simulink model "model"  (R2017b)
settings: Solver=ode45  StartTime=0.0  StopTime=0.05  RelTol=1e-3  EnableMultiTasking=on
InitFcn:
  | Fs=100e3;
  | w=Fs*2*pi;
  | 
  | Vdc=100;
  | 
  | LP=200e-6;
  | LS=LP;
  | 
  | CP=1/w^2/LP;
  | CS=1/w^2/LS;
  | 
  | MPS=20e-6;
  | 
  | 
  | Rlp=0.1;
  | Rls=0.1;
undefined symbols (not defined in the file): LM, MPM, MSM, Rlm
libraries: powerlib x20, simulink x2, peRmsMeasurement x1
settings Model: Creator=User  LastModifiedBy=SuperWindows
settings DataIOCC: LimitDataPoints=on  SaveFormat=Array
settings OptimizationCC: LifeSpan=inf
settings DebuggingCC: SolverPrmCheckMsg=warning  SFUnexpectedBacktrackingDiag=warning  SFNoUnconditionalDefaultTransitionDiag=warning  SFExecutionAtInitializationDiag=none
settings HardwareCC: ProdBitPerPointer=32  ProdBitPerSizeT=32  ProdBitPerPtrDiffT=32  ProdLargestAtomicFloat=None  ProdIntDivRoundTo=Undefined  ProdEndianess=Unspecified  ProdWordSize=32  ProdHWDeviceType=32-bit Generic
settings ModelReferenceCC: PropagateSignalLabelsOutOfModel=off
settings CodeAppCC: StateflowObjectComments=on
settings GRTTargetCC: TargetLangStandard=C89/C90 (ANSI)  GeneratePreprocessorConditionals=Disable all
settings ConfigComp: CovMetricSettings=dw  CovHtmlReporting=on  CovSaveCumulativeToWorkspaceVar=on  CovSaveSingleToWorkspaceVar=on  CovExternalEMLEnable=off  CovSFcnEnable=off
settings SimscapeCC: SimscapeNormalizeSystem=off

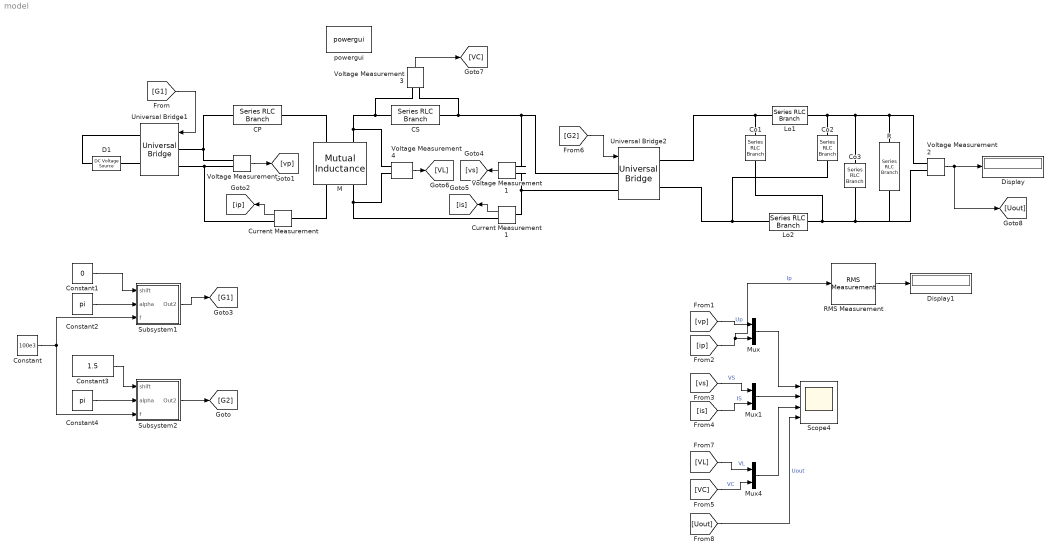
== system model ==
  CP : powerlib/Elements/Series RLC Branch  LConnTagsString=__new0  RConnTagsString=__new0  BranchType=C  Resistance=5  Inductance=1e-3  SetiL0=off  InitialCurrent=0  Capacitance=CP  Setx0=off  InitialVoltage=0  Measurements=Branch voltage
  CS : powerlib/Elements/Series RLC Branch  LConnTagsString=__new0  RConnTagsString=__new0  BranchType=C  Resistance=1  Inductance=1e-3  SetiL0=off  InitialCurrent=0  Capacitance=CS  Setx0=off  InitialVoltage=0  Measurements=Branch voltage
  Co1 : powerlib/Elements/Series RLC Branch  LConnTagsString=__new0  RConnTagsString=__new0  BranchType=C  Resistance=1  Inductance=1e-3  SetiL0=off  InitialCurrent=0  Capacitance=4700e-6  Setx0=on  InitialVoltage=60  Measurements=Branch voltage
  Co2 : powerlib/Elements/Series RLC Branch  LConnTagsString=__new0  RConnTagsString=__new0  BranchType=C  Resistance=1  Inductance=1e-3  SetiL0=off  InitialCurrent=0  Capacitance=4700e-6  Setx0=on  InitialVoltage=60  Measurements=Branch voltage
  Co3 : powerlib/Elements/Series RLC Branch  LConnTagsString=__new0  RConnTagsString=__new0  BranchType=C  Resistance=1  Inductance=1e-3  SetiL0=off  InitialCurrent=0  Capacitance=4700e-6  Setx0=on  InitialVoltage=60  Measurements=Branch voltage
  Constant : Constant  Value=100e3
  Constant1 : Constant  Value=0
  Constant2 : Constant  Value=pi
  Constant3 : Constant  Value=1.5
  Constant4 : Constant  Value=pi
  Current Measurement : powerlib/Measurements/Current Measurement  PhasorSimulation=off  OutputType=Complex  PSBequivalent=0
  Current Measurement1 : powerlib/Measurements/Current Measurement  PhasorSimulation=off  OutputType=Complex  PSBequivalent=0
  D1 : powerlib/Electrical Sources/DC Voltage Source  Amplitude=Vdc  Measurements=None
  Display : Display
  Display1 : Display
  Lo1 : powerlib/Elements/Series RLC Branch  LConnTagsString=__new0  RConnTagsString=__new0  BranchType=L  Resistance=1  Inductance=1e-3  SetiL0=off  InitialCurrent=0  Capacitance=4700e-6  Setx0=on  InitialVoltage=60  Measurements=Branch voltage
  Lo2 : powerlib/Elements/Series RLC Branch  LConnTagsString=__new0  RConnTagsString=__new0  BranchType=L  Resistance=1  Inductance=1e-3  SetiL0=off  InitialCurrent=0  Capacitance=4700e-6  Setx0=on  InitialVoltage=60  Measurements=Branch voltage
  M : powerlib/Elements/Mutual Inductance  LConnTagsString=a|b  RConnTagsString=A|B  TypeOfMutual=Two or three windings with equal mutual terms  NumberOfWindings=3  SelfImpedance1=[Rlp LP]  SelfImpedance2=[Rls LS]  ThreeWindings=off  SelfImpedance3=[ 1.1 1.1e-03]  MutualImpedance=[0.0 MPS]  InductanceMatrix="[LP MPS  MPM ;  MPS LS  MSM;  MPM MSM LM ]"  ResistanceMatrix="[Rlp 0  0 ;  0 Rls  0;  0 0 Rlm ]"  Measurements=None
      settings: AttributesFormatString=\n  SourceProductName=Simscape Power Systems  SourceProductBaseCode=PS
  Mux : Mux  Inputs=2
  Mux1 : Mux  Inputs=2
  Mux4 : Mux  Inputs=2
  R : powerlib/Elements/Series RLC Branch  LConnTagsString=__new0  RConnTagsString=__new0  BranchType=R  Resistance=10  Inductance=1e-3  SetiL0=off  InitialCurrent=0  Capacitance=CS  Setx0=off  InitialVoltage=0  Measurements=None
  RMS Measurement : peRmsMeasurement/RMS Measurement  OverrideUsingVariant=Total  F=Fs  SpecifyHarmonics=off  K=[0 1 2]  Ts=1/Fs/100
  Scope4 : Scope  NumInputPorts=4
  Subsystem1 : Subsystem  mask{f=Fs}
  Subsystem2 : Subsystem  mask{f=Fs}
  Universal Bridge1 : powerlib/Power Electronics/Universal Bridge  Arms=2  SnubberResistance=1e5  SnubberCapacitance=inf  Device=MOSFET / Diodes  Ron=1e-3  Lon=0  ForwardVoltages="[  0  0  ]"  ForwardVoltage=0  GTOparameters=[ 10e-6 , 20e-6 ]  IGBTparameters=[ 1e-6 , 2e-6 ]  Measurements=None  Measurements_2=None  converterType=Rectifier
  Universal Bridge2 : powerlib/Power Electronics/Universal Bridge  Arms=2  SnubberResistance=1e5  SnubberCapacitance=inf  Device=MOSFET / Diodes  Ron=1e-3  Lon=0  ForwardVoltages="[  0  0  ]"  ForwardVoltage=0  GTOparameters=[ 10e-6 , 20e-6 ]  IGBTparameters=[ 1e-6 , 2e-6 ]  Measurements=None  Measurements_2=None  converterType=Rectifier
  Voltage Measurement{,1..4} (5 alike) : powerlib/Measurements/Voltage Measurement  PhasorSimulation=off  OutputType=Complex  PSBequivalent=0
  powergui : powerlib/powergui  Priority=1  SimulationMode=Discrete  SampleTime=1e-8  frequency=60  Iterations=50  frequencyindice=0  Pbase=100e6  ErrMax=1e-4  UnitsV=kV  UnitsW=MW  buscounter=0  FunctionMessages=off  echomessages=off  EnableUseOfTLC=off  CurrentSourceSwitches=off  DisableSnubberDevices=off  DisableRonSwitches=off  DisableVfSwitches=off  DisplayEquations=off  SolverType=Tustin  Interpol=off  ExternalGateDelay=off  methode=off  Ts=0  x0status=blocks  SPID=off  SwTol=0  HookPort=off  RestoreLinks=warning  ResistiveCurrentMeasurement=off  Frange=[0:2:500]  Ylog=off  Xlog=on  ShowGrid=off  save=off  variable=ZData  structure=0  ZoomFFT=off  StartTime=0.0  cycles=1  DisplayStyle=1  fundamental=60  FreqAxis=off  MaxFrequency=1000  frequencyindicesteady=1  RmsSteady=1  display=off
  wires:
  Subsystem1/1(Out2) -> [G1]
  [G1] -> Universal Bridge1/1
  Voltage Measurement/1 -> [vp]
  Current Measurement/1 -> [ip]
  Voltage Measurement1/1 -> [vs]
  Current Measurement1/1 -> [is]
  [vp] -> Mux/1  "Up"
  [ip] -> RMS Measurement/1, Mux/2  "Ip"
  [vs] -> Mux1/1  "VS"
  [is] -> Mux1/2  "IS"
  Voltage Measurement2/1 -> [Uout], Display/1
  Constant1/1 -> Subsystem1/1(shift)
  [G2] -> Universal Bridge2/1
  Constant2/1 -> Subsystem1/2("alpha ")
  Constant4/1 -> Subsystem2/2("alpha ")
  Constant3/1 -> Subsystem2/1(shift)
  Subsystem2/1(Out2) -> [G2]
  Mux1/1 -> Scope4/2
  Voltage Measurement4/1 -> [VL]
  Voltage Measurement3/1 -> [VC]
  [VL] -> Mux4/1  "VL"
  [VC] -> Mux4/2  "VC"
  Mux/1 -> Scope4/1
  Mux4/1 -> Scope4/3
  [Uout] -> Scope4/4  "Uout"
  Constant/1 -> Subsystem1/3(f), Subsystem2/3(f)
  RMS Measurement/1 -> Display1/1
  connections:
  D1/RConn1 -- Universal Bridge1/RConn1
  D1/LConn1 -- Universal Bridge1/RConn2
  Universal Bridge1/LConn1 -- Voltage Measurement/LConn1 -- CP/LConn1
  CP/RConn1 -- M/LConn1
  Voltage Measurement1/LConn1 -- CS/RConn1 -- Voltage Measurement3/LConn1 -- Universal Bridge2/LConn1
  Voltage Measurement2/LConn2 -- R/RConn1 -- Co3/RConn1 -- Co1/RConn1 -- Lo2/RConn1
  Current Measurement/LConn1 -- M/RConn1
  Current Measurement/RConn1 -- Universal Bridge1/LConn2 -- Voltage Measurement/LConn2
  Current Measurement1/RConn1 -- Voltage Measurement4/LConn2 -- M/RConn2
  Voltage Measurement1/LConn2 -- Current Measurement1/LConn1 -- Universal Bridge2/LConn2
  Voltage Measurement2/LConn1 -- R/LConn1 -- Co3/LConn1 -- Lo1/RConn1 -- Co2/LConn1
  Voltage Measurement3/LConn2 -- CS/LConn1 -- Voltage Measurement4/LConn1 -- M/LConn2
  Lo1/LConn1 -- Universal Bridge2/RConn1 -- Co1/LConn1
  Lo2/LConn1 -- Co2/RConn1 -- Universal Bridge2/RConn2

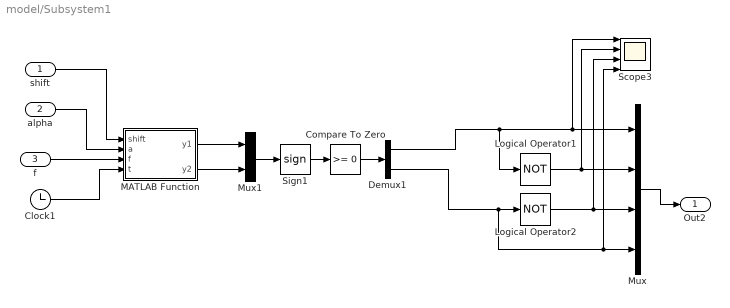
== system model/Subsystem1 ==
  shift : Inport
  "alpha " : Inport  Port=2
  f : Inport  Port=3
  Clock1 : Clock
  Compare To Zero : simulink/Logic and Bit Operations/Compare To Zero  relop=>=  OutDataTypeStr=boolean
  Demux1 : Demux  Outputs=2
  Logical Operator1 : Logic  Operator=NOT  AllPortsSameDT=off  OutDataTypeStr=boolean
  Logical Operator2 : Logic  Operator=NOT  AllPortsSameDT=off  OutDataTypeStr=boolean
  MATLAB Function : MATLAB Function  TreatAsAtomicUnit=on
  Mux : Mux
  Mux1 : Mux  Inputs=2
  Scope3 : Scope  NumInputPorts=4
  Sign1 : Signum
  Out2 : Outport
  wires:
  "alpha "/1 -> MATLAB Function/2(a)
  Clock1/1 -> MATLAB Function/4(t)
  MATLAB Function/1(y1) -> Mux1/1
  Logical Operator1/1 -> Scope3/2, Mux/2
  Mux/1 -> Out2/1
  MATLAB Function/2(y2) -> Mux1/2
  Mux1/1 -> Sign1/1
  Sign1/1 -> Compare To Zero/1
  Compare To Zero/1 -> Demux1/1
  Demux1/1 -> Scope3/1, Mux/1, Logical Operator1/1
  Demux1/2 -> Mux/4, Scope3/4, Logical Operator2/1
  Logical Operator2/1 -> Scope3/3, Mux/3
  shift/1 -> MATLAB Function/1(shift)
  f/1 -> MATLAB Function/3(f)

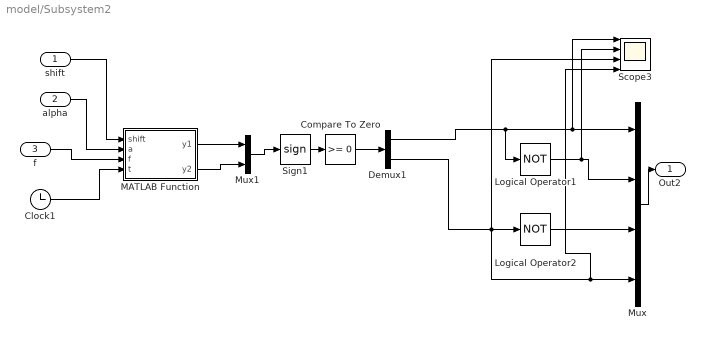
== system model/Subsystem2 ==
  shift : Inport
  "alpha " : Inport  Port=2
  f : Inport  Port=3
  Clock1 : Clock
  Compare To Zero : simulink/Logic and Bit Operations/Compare To Zero  relop=>=  OutDataTypeStr=boolean
  Demux1 : Demux  Outputs=2
  Logical Operator1 : Logic  Operator=NOT  AllPortsSameDT=off  OutDataTypeStr=boolean
  Logical Operator2 : Logic  Operator=NOT  AllPortsSameDT=off  OutDataTypeStr=boolean
  MATLAB Function : MATLAB Function  TreatAsAtomicUnit=on
  Mux : Mux
  Mux1 : Mux  Inputs=2
  Scope3 : Scope  NumInputPorts=4
  Sign1 : Signum
  Out2 : Outport
  wires:
  "alpha "/1 -> MATLAB Function/2(a)
  Clock1/1 -> MATLAB Function/4(t)
  MATLAB Function/1(y1) -> Mux1/1
  Logical Operator1/1 -> Scope3/2, Mux/2
  Mux/1 -> Out2/1
  MATLAB Function/2(y2) -> Mux1/2
  Mux1/1 -> Sign1/1
  Sign1/1 -> Compare To Zero/1
  Compare To Zero/1 -> Demux1/1
  Demux1/1 -> Logical Operator1/1, Scope3/1, Mux/1
  Demux1/2 -> Scope3/3, Logical Operator2/1, Scope3/4, Mux/4
  Logical Operator2/1 -> Mux/3
  shift/1 -> MATLAB Function/1(shift)
  f/1 -> MATLAB Function/3(f)

== matlab function model/Subsystem1/MATLAB Function ==
  data: shift input; y1 output; a input; f input; t input; y2 output
function [y1,y2] = fcn(shift,a,f,t)
w=2*pi*f;
y1 = sin(w*t-a/2+shift);
y2 = sin(w*t-pi+a/2+shift);
%#codegen

== matlab function model/Subsystem2/MATLAB Function ==
  data: shift input; y1 output; a input; f input; t input; y2 output
function [y1,y2] = fcn(shift,a,f,t)
w=2*pi*f;
y1 = sin(w*t-a/2+shift);
y2 = sin(w*t-pi+a/2+shift);
%#codegen
